simulink model "Main_simulation_optimised_BATTERYonly"  (R2017b)
settings: Solver=FixedStepDiscrete  StartTime=0  StopTime=20  RelTol=1e-3  EnableMultiTasking=on
PreLoadFcn:
  | Ts=2e-6;
undefined symbols (not defined in the file): DiscIntNeverNeededParam, Ion, Lithium, sigbuilder_block
libraries: powerlib x20, electricdrivelib x5, autolibshared x5, powerlib_meascontrol x3, sdolib x2, spsDrivesDcBusModel x1, spsDrivesPrivateModels x1, spsDrivesOutputSelector x1, spsDrivesSpeedControllerModel x1, simulink x1
(part 2 of 2)

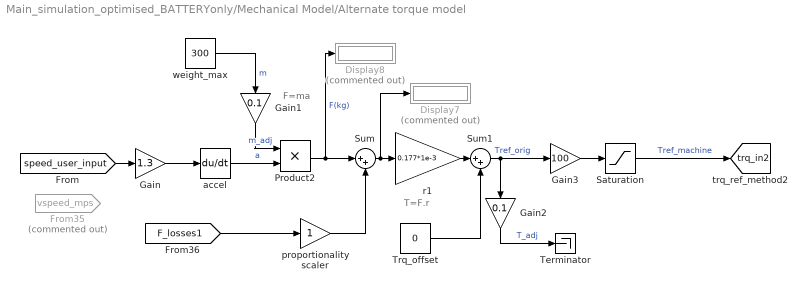
== system Main_simulation_optimised_BATTERYonly/Mechanical Model/Alternate torque model ==
  note: T=F.r
  note: F=ma
  Display7 : Display  Commented=on
  Display8 : Display  Commented=on
  From35 : From  Commented=on  GotoTag=vspeed_mps  TagVisibility=global
  Gain : Gain  Gain=1.3
  Gain1 : Gain  Gain=0.1
  Gain2 : Gain  Gain=0.1
  Gain3 : Gain  Gain=100
  Product2 : Product
  Saturation : Saturate  UpperLimit=22  LowerLimit=-30
  Sum : Sum  Inputs=|++
  Sum1 : Sum  Inputs=|++
  Terminator : Terminator
  Trq_offset : Constant  Value=0
  accel : Derivative
  proportionality scaler : Gain
  r1 : Gain  Gain=0.177*1e-3
  weight_max : Constant  Value=300
  tag scope: trq_in2=global
  wires:
  weight_max/1 -> Gain1/1  "m"
  accel/1 -> Product2/2  "a"
  [speed_user_input] -> Gain/1
  [F_losses1] -> proportionality scaler/1
  Product2/1 -> Display8/1, Sum/1  "F(kg)"
  Sum1/1 -> Gain2/1, Gain3/1  "Tref_orig"
  Sum/1 -> Display7/1, r1/1
  r1/1 -> Sum1/1
  Trq_offset/1 -> Sum1/2
  Gain/1 -> accel/1
  proportionality scaler/1 -> Sum/2
  Gain1/1 -> Product2/1  "m_adj"
  Gain2/1 -> Terminator/1  "T_adj"
  Saturation/1 -> [trq_in2]  "Tref_machine"
  Gain3/1 -> Saturation/1

== system Main_simulation_optimised_BATTERYonly/Mechanical Model/Gradient generator ==
  Demux : Demux  Tag=STV Demux  Outputs=1
  FromWs : FromWorkspace  Tag=STV FromWs  VariableName=tuvar  SampleTime=0
      SigBuilderData=|
      | common.afterFinalStr = 'Extrapolate'
      | common.sampleTime = 0
      | dataSet.timeRange = [0 10]
      | dataSet.name = 'Group 1'
      | sbobj.Groups.Name = 'Group 1'
      | sbobj.Groups.Signals.Name = 'Gradient'
      | sbobj.Groups.Signals.XData = [0 1 1.2 2.6 2.8 3.8 5 5.5 6.62 7.16 10]
      | sbobj.Groups.Signals.YData = [0 1 5 5 1.96 0.3 0.25 -2.2 -2.2 0 0]
  Gradient : Outport  Tag=STV Outport
  wires:
  FromWs/1 -> Demux/1
  Demux/1 -> Gradient/1

== system Main_simulation_optimised_BATTERYonly/Mechanical Model/Signal Builder ==
  Demux : Demux  Tag=STV Demux  Outputs=1
  FromWs : FromWorkspace  Tag=STV FromWs  VariableName=tuvar  SampleTime=0
      SigBuilderData=|
      | common.afterFinalStr = 'Extrapolate'
      | common.sampleTime = 0
      | dataSet.timeRange = [0 10]
      | dataSet.name = 'Group 1'
      | sbobj.Groups.Name = 'Group 1'
      | sbobj.Groups.Signals.Name = 'Signal 2'
      | sbobj.Groups.Signals.XData = [0 1 1 2 2 2.39 2.39 3.81 5 5 6.45 6.45 6.8 6.8 8 8 9 9 10]
      | sbobj.Groups.Signals.YData = [0 5.1 0.2 11 7.5 2.4 0.6 7.1 1.2 0.4 8.7 7.7 14.7 13 13.2 11.3 7.1 0.2 0.2]
  Signal 2 : Outport  Tag=STV Outport
  wires:
  FromWs/1 -> Demux/1
  Demux/1 -> Signal 2/1

== system Main_simulation_optimised_BATTERYonly/Mechanical Model/Torque model 1 -- redacted ==
  note: torque reference generation
  note: real torque gain factor - 0.1
      | for simulation - 0.01
  Abs : Abs
  Product1 : Product  Inputs=4
  Saturation1 : Saturate  UpperLimit=15  LowerLimit=-15
  Saturation2 : Saturate  UpperLimit=30  LowerLimit=-40
  torque gain : Constant  Value=5
  tag scope: torque_input=global
  wires:
  Saturation1/1 -> Product1/2
  Abs/1 -> Product1/3
  [acc_dec_rate] -> Saturation1/1
  Saturation2/1 -> [torque_input]  "trq_input"
  Product1/1 -> Saturation2/1
  torque gain/1 -> Product1/4
  [speed_ref] -> Product1/1
  [ad_detect] -> Abs/1

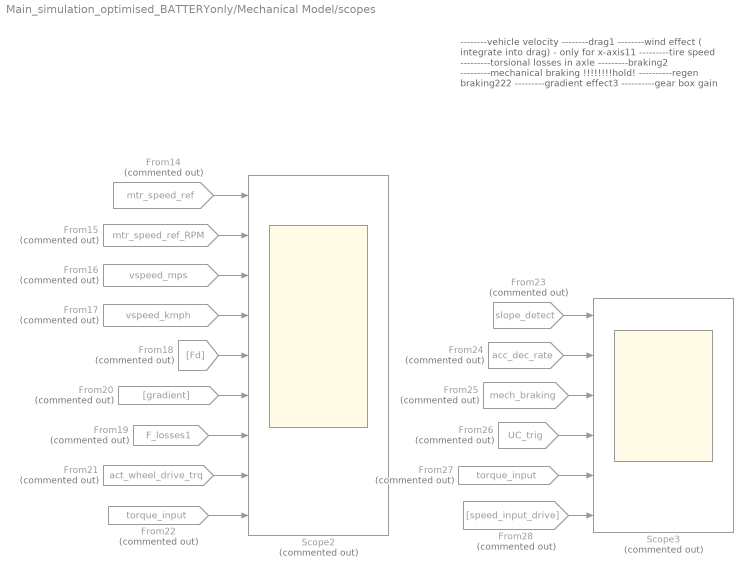
== system Main_simulation_optimised_BATTERYonly/Mechanical Model/scopes ==
  note: --------vehicle velocity
      |
      | --------drag1
      |
      | --------wind effect ( integrate into drag) - only for x-axis11
      |
      | ---------tire speed
      |
      | ---------torsional losses in axle
      |
      | ---------braking2
      |
      | ---------mechanical braking !!!!!!!!hold!
      |
      | ----------regen braking222
      |
      | ---------gradient effect3
      |
      | ----------gear box gain
  From14 : From  Commented=on  GotoTag=mtr_speed_ref  TagVisibility=global
  From15 : From  Commented=on  GotoTag=mtr_speed_ref_RPM  TagVisibility=global
  From16 : From  Commented=on  GotoTag=vspeed_mps  TagVisibility=global
  From17 : From  Commented=on  GotoTag=vspeed_kmph  TagVisibility=global
  From18 : From  Commented=on  GotoTag=Fd
  From19 : From  Commented=on  GotoTag=F_losses1  TagVisibility=global
  From20 : From  Commented=on  GotoTag=gradient
  From21 : From  Commented=on  GotoTag=act_wheel_drive_trq  TagVisibility=global
  From22 : From  Commented=on  GotoTag=torque_input  TagVisibility=global
  From23 : From  Commented=on  GotoTag=slope_detect  TagVisibility=global
  From24 : From  Commented=on  GotoTag=acc_dec_rate  TagVisibility=global
  From25 : From  Commented=on  GotoTag=mech_braking  TagVisibility=global
  From26 : From  Commented=on  GotoTag=UC_trig  TagVisibility=global
  From27 : From  Commented=on  GotoTag=torque_input  TagVisibility=global
  From28 : From  Commented=on  GotoTag=speed_input_drive
  Scope2 : Scope  Commented=on  NumInputPorts=9
  Scope3 : Scope  Commented=on  NumInputPorts=6
  wires:
  From28/1 -> Scope3/6
  From14/1 -> Scope2/1
  From24/1 -> Scope3/2
  From15/1 -> Scope2/2
  From26/1 -> Scope3/4
  From25/1 -> Scope3/3
  From27/1 -> Scope3/5
  From23/1 -> Scope3/1
  From16/1 -> Scope2/3
  From20/1 -> Scope2/6
  From17/1 -> Scope2/4
  From22/1 -> Scope2/9
  From19/1 -> Scope2/7
  From21/1 -> Scope2/8
  From18/1 -> Scope2/5

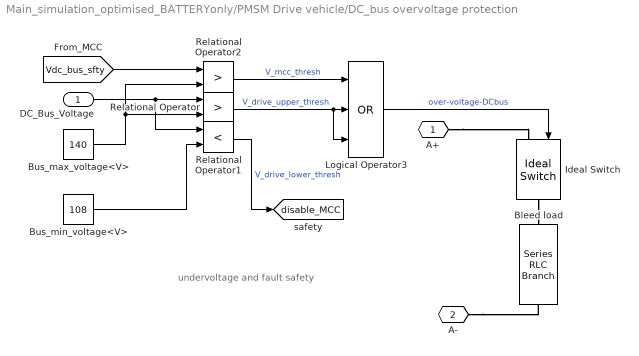
== system Main_simulation_optimised_BATTERYonly/PMSM Drive vehicle/DC_bus overvoltage protection ==
  note: undervoltage and fault safety
  DC_Bus_Voltage : Inport
  Bleed load : powerlib/Elements/Series RLC Branch  LConnTagsString=__new0  RConnTagsString=__new0  BranchType=RL  Resistance=2  Inductance=5e-6  SetiL0=off  InitialCurrent=0  Capacitance=1e-6  Setx0=off  InitialVoltage=0  Measurements=None
  Bus_max_voltage<V> : Constant  Value=140
  Bus_min_voltage<V> : Constant  Value=108
  Ideal Switch : powerlib/Power Electronics/Ideal Switch  Ron=0.001  Lon=0  IC=0  Rs=10e3  Cs=1e-6  Measurements=off
  Logical Operator3 : Logic  Operator=OR  Inputs=3  AllPortsSameDT=off  OutDataTypeStr=boolean
  Relational Operator : RelationalOperator  Operator=>  OutDataTypeStr=boolean  RndMeth=Simplest
  Relational Operator1 : RelationalOperator  Operator=<  OutDataTypeStr=boolean  RndMeth=Simplest
  Relational Operator2 : RelationalOperator  Operator=>  OutDataTypeStr=boolean  RndMeth=Simplest
  A+ : PMIOPort  Port=1  Side=Left
  A- : PMIOPort  Port=2  Side=Left
  tag scope: disable_MCC=global
  wires:
  DC_Bus_Voltage/1 -> Relational Operator1/1, Relational Operator/1
  Relational Operator/1 -> Logical Operator3/3, Logical Operator3/2  "V_drive_upper_thresh"
  Bus_min_voltage<V>/1 -> Relational Operator1/2
  Logical Operator3/1 -> Ideal Switch/1  "over-voltage-DCbus"
  Bus_max_voltage<V>/1 -> Relational Operator2/2, Relational Operator/2
  [Vdc_bus_sfty] -> Relational Operator2/1
  Relational Operator2/1 -> Logical Operator3/1  "V_mcc_thresh"
  Relational Operator1/1 -> [disable_MCC]  "V_drive_lower_thresh"
  connections:
  Ideal Switch/RConn1 -- Bleed load/LConn1
  A+/RConn1 -- Ideal Switch/LConn1
  A-/RConn1 -- Bleed load/RConn1

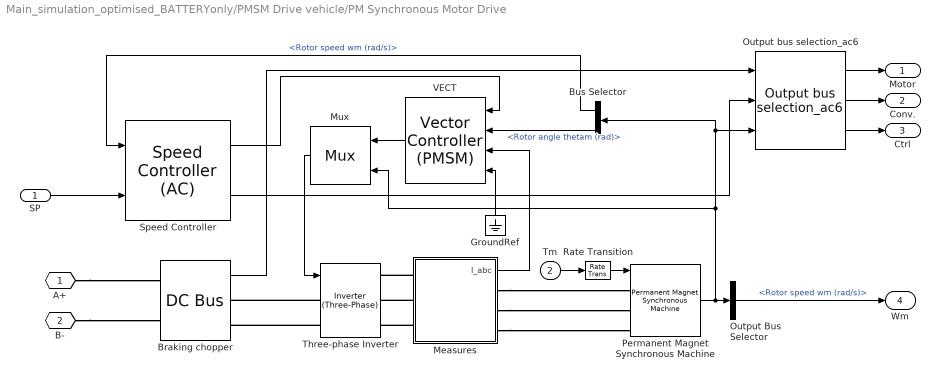
== system Main_simulation_optimised_BATTERYonly/PMSM Drive vehicle/PM Synchronous Motor Drive ==
  SP : Inport
  Tm : Inport  Port=2
  Braking chopper : spsDrivesDcBusModel/DC Bus   busType=Capacitive (generic)  Ts=baseSampleTime  capacitance=cap_bus  inductance=0  Setx0=off  InitialVoltage=600  Rbrake=Rbrake  frequency=fbrake  activationVoltage=activationVoltage  shutdownVoltage=shutdownVoltage
      settings: SourceProductName=The database C:\Users\ak23510\AppData\Roaming\MathWorks\MATLAB\R2017a\slblocks_master.db is locked, or a table in the database is locked. (database is locked)
  Bus Selector : BusSelector  OutputSignals=Rotor speed wm (rad/s),Rotor angle thetam (rad)
  GroundRef : Ground
  Measures : Subsystem
  Mux : spsDrivesPrivateModels/Mux  OverrideUsingVariant=Detailed  detailLevel=Detailed  driveType=AC6
      settings: AttributesFormatString=%<BlockChoice>  SourceProductName=The database C:\Users\ak23510\AppData\Roaming\MathWorks\MATLAB\R2017a\slblocks_master.db is locked, or a table in the database is locked. (database is locked)
  Output Bus Selector : BusSelector  OutputSignals=Rotor speed wm (rad/s)
  Output bus selection_ac6 : spsDrivesOutputSelector/Output bus selection_ac6  OverrideUsingVariant=Multiple_output_buses
      settings: AttributesFormatString=%<BlockChoice>  SourceProductName=The database C:\Users\ak23510\AppData\Roaming\MathWorks\MATLAB\R2017a\slblocks_master.db is locked, or a table in the database is locked. (database is locked)
  Permanent Magnet Synchronous Machine : powerlib/Machines/Permanent Magnet Synchronous Machine  NbPhases=3  FluxDistribution=Sinusoidal  RotorType=Salient-pole  MechanicalLoad=Torque Tm  PresetModel=No  ShowDetailedParameters=on  MeasurementBus=off  Resistance=Rs  Inductance=0  dqInductances=[Lls,Lms]  La=0.000835  MachineConstant=Flux linkage established by magnets (V.s)  Flux=0.175  VoltageCst=126.966  TorqueCst=1.05  Flat=0  Mechanical=[J,Friction,p]  PolePairs=4  InitialConditions=[wm,thetam,ia,ib]  InitialConditions5ph=[0 0 0 0 0 0]  TsPowergui=0  TsBlock=-1  RefAngle=90 degrees behind phase A axis (modified Park)
      settings: AttributesFormatString=\n  SourceProductName=Simscape Power Systems
  Rate Transition : RateTransition  OutPortSampleTime=baseSampleTime
  Speed Controller : spsDrivesSpeedControllerModel/Speed Controller (AC)  OverrideUsingVariant=AC345  ctrlType=Without flux reference output  SwK=Speed regulation  Ts=baseSampleTime  ramp=[Dec,Acc]  kp=kp_sc  ki=ki_sc  fc=fc_sc  ctrl_sat=[Tmin,Tmax]  Tsc=Tsc  fn=60  p=2  nf=0.3
      settings: SourceProductName=The database C:\Users\ak23510\AppData\Roaming\MathWorks\MATLAB\R2017a\slblocks_master.db is locked, or a table in the database is locked. (database is locked)
  Three-phase Inverter : electricdrivelib/Fundamental Drive Blocks/Inverter (Three-Phase)  OverrideUsingVariant=Detailed  detailLevel=Detailed  driveType=PMSM vector control  Ts=baseSampleTime  SnubberResistance=Rsnb_inv  SnubberCapacitance=Csnb_inv  Device=IGBT / Diodes  Ron=Ron_inv  ForwardVoltages="[  Vf_inv  Vfd_inv  ]"  GTOparameters=[Tf_GTO,Tt_GTO]  IGBTparameters="[  Tf  Tt  ]"  Measurements=All voltages and currents  converterType=Inverter  SourceFrequency=sourceFrequency  ReferenceFrame=Rotor  dqInductances=[Lls,Lms]  Inductance=0  Ls=0  Resistance=Rs  Flux=FluxCst  Stator_sm=[2.01e-3,4.289e-4,4.477e-3,1.354e-3]  Stator_im=[14.85e-3,0.3027e-3]  Rotor=[9.295e-3,0.3027e-3]  Lm=10.46e-3  p=p
      settings: AttributesFormatString=%<BlockChoice>  SourceProductName=Simscape Power Systems  SourceProductBaseCode=PS
  VECT : electricdrivelib/Fundamental Drive Blocks/Vector Controller (PMSM)  OverrideUsingVariant=Detailed_3ph  detailLevel=Detailed  nb_ph=3  modulationType=Hysteresis  Ts_vect=Tvect  h=h  freq_max=freq_max  fc_bus=fc_bus  car_freq=car_freq  nb_p=p  machineConstant=Flux linkage established by magnets (V.s)  fluxConstant=FluxCst  voltageConstant=VoltageCst  torqueConstant=TorqueCst  kp_Id=kp_Id  ki_Id=ki_Id  kp_Iq=kp_Iq  ki_Iq=ki_Iq
      settings: AttributesFormatString=%<BlockChoice>  SourceProductName=Simscape Power Systems  SourceProductBaseCode=PS
  A+ : PMIOPort  Port=1  Side=Left
  B- : PMIOPort  Port=2  Side=Left
  Motor : Outport
  Conv. : Outport  Port=2
  Ctrl : Outport  Port=3
  Wm : Outport  Port=4
  wires:
  Mux/1 -> Three-phase Inverter/1
  Speed Controller/1 -> VECT/1
  Output bus selection_ac6/1 -> Motor/1
  Output bus selection_ac6/3 -> Ctrl/1
  Output bus selection_ac6/2 -> Conv./1
  Rate Transition/1 -> Permanent Magnet Synchronous Machine/1
  Tm/1 -> Rate Transition/1
  Output Bus Selector/1 -> Wm/1  "<Rotor speed wm (rad/s)>"
  Braking chopper/1 -> Output bus selection_ac6/1
  SP/1 -> Speed Controller/2
  Permanent Magnet Synchronous Machine/1 -> Output Bus Selector/1, Mux/2, Output bus selection_ac6/3, Bus Selector/1
  Measures/1(I_abc) -> VECT/3
  Speed Controller/2 -> Output bus selection_ac6/2
  VECT/1 -> Mux/1
  Bus Selector/1 -> Speed Controller/1  "<Rotor speed wm (rad/s)>"
  Bus Selector/2 -> VECT/2  "<Rotor angle thetam (rad)>"
  GroundRef/1 -> VECT/4
  connections:
  Three-phase Inverter/LConn2 -- Braking chopper/RConn2
  Three-phase Inverter/LConn1 -- Braking chopper/RConn1
  B-/RConn1 -- Braking chopper/LConn2
  A+/RConn1 -- Braking chopper/LConn1
  Measures/RConn1 -- Permanent Magnet Synchronous Machine/LConn1
  Measures/RConn2 -- Permanent Magnet Synchronous Machine/LConn2
  Measures/RConn3 -- Permanent Magnet Synchronous Machine/LConn3
  Measures/LConn1 -- Three-phase Inverter/RConn1
  Measures/LConn2 -- Three-phase Inverter/RConn2
  Measures/LConn3 -- Three-phase Inverter/RConn3

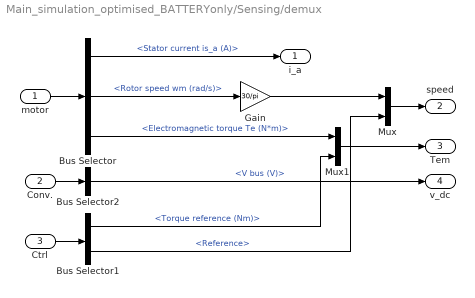
== system Main_simulation_optimised_BATTERYonly/Sensing/demux ==
  motor : Inport
  Conv. : Inport  Port=2
  Ctrl : Inport  Port=3
  Bus Selector : BusSelector  OutputSignals=Stator current is_a (A),Rotor speed wm (rad/s),Electromagnetic torque Te (N*m)
  Bus Selector1 : BusSelector  OutputSignals=Torque reference (Nm),Reference
  Bus Selector2 : BusSelector  OutputSignals=V bus (V)
  Gain : Gain  Gain=30/pi  SaturateOnIntegerOverflow=on  OutDataTypeStr=Inherit: Same as input  ParamDataTypeStr=Inherit: Same as input
  Mux : Mux  Inputs=2
  Mux1 : Mux  Inputs=2
  i_a : Outport
  speed : Outport  Port=2
  Tem : Outport  Port=3
  v_dc : Outport  Port=4
  wires:
  Bus Selector/2 -> Gain/1  "<Rotor speed wm (rad/s)>"
  Bus Selector2/1 -> v_dc/1  "<V bus (V)>"
  Conv./1 -> Bus Selector2/1
  Ctrl/1 -> Bus Selector1/1
  Bus Selector1/1 -> Mux1/2  "<Torque reference (Nm)>"
  Bus Selector1/2 -> Mux/2  "<Reference>"
  Gain/1 -> Mux/1
  Bus Selector/1 -> i_a/1  "<Stator current is_a (A)>"
  Bus Selector/3 -> Mux1/1  "<Electromagnetic torque Te (N*m)>"
  Mux1/1 -> Tem/1
  Mux/1 -> speed/1
  motor/1 -> Bus Selector/1

== system Main_simulation_optimised_BATTERYonly/PMSM Drive vehicle/PM Synchronous Motor Drive/Measures ==
  Current Measurement : powerlib/Measurements/Current Measurement  Tag=PoWeRsYsTeMmEaSuReMeNt  PhasorSimulation=off  OutputType=Magnitude  PSBequivalent=0
  Current Measurement1 : powerlib/Measurements/Current Measurement  Tag=PoWeRsYsTeMmEaSuReMeNt  PhasorSimulation=off  OutputType=Magnitude  PSBequivalent=0
  Current Measurement2 : powerlib/Measurements/Current Measurement  Tag=PoWeRsYsTeMmEaSuReMeNt  PhasorSimulation=off  OutputType=Magnitude  PSBequivalent=0
  Mux1 : Mux  Inputs=3
  Ta : PMIOPort  Port=1  Side=Left
  Tb : PMIOPort  Port=2  Side=Left
  Tc : PMIOPort  Port=3  Side=Left
  Mta : PMIOPort  Port=4  Side=Right
  Mtb : PMIOPort  Port=5  Side=Right
  Mtc : PMIOPort  Port=6  Side=Right
  I_abc : Outport
  wires:
  Current Measurement1/1 -> Mux1/2
  Current Measurement/1 -> Mux1/1
  Current Measurement2/1 -> Mux1/3
  Mux1/1 -> I_abc/1
  connections:
  Current Measurement1/RConn1 -- Mtb/RConn1
  Tb/RConn1 -- Current Measurement1/LConn1
  Current Measurement/RConn1 -- Mta/RConn1
  Ta/RConn1 -- Current Measurement/LConn1
  Tc/RConn1 -- Current Measurement2/LConn1
  Current Measurement2/RConn1 -- Mtc/RConn1
